simulink model "DC_Motor"  (R2023b)
settings: Solver=VariableStepAuto  StartTime=0.0  StopTime=20  RelTol=1e-3
undefined symbols (not defined in the file): Custom_PID

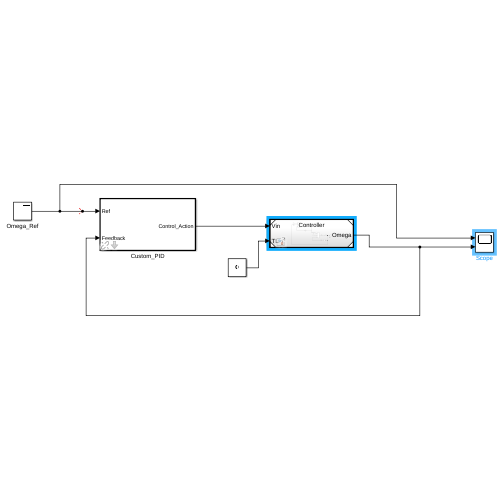
[thumbnail: Simulink's stored preview of the top-level diagram]
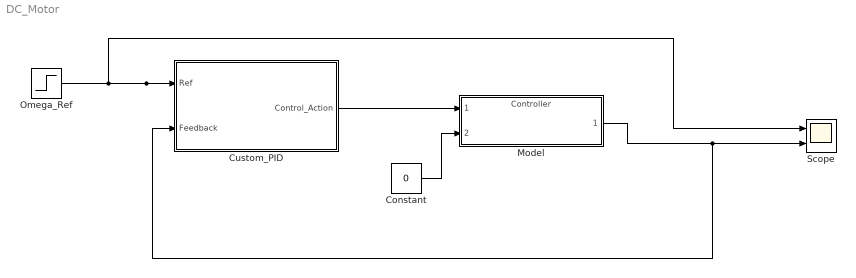
== system DC_Motor ==
  Constant : Constant  Value=0
  Custom_PID : Subsystem  AncestorBlock=Custom_PID/Custom_PID  TreatAsAtomicUnit=on  mask{Kp=8, Ki=2.5, Kd=2, IC=0}
      mask prompts: Kp "Proportional"; Ki "Integral"; Kd "Differential"; IC "Initial Condition"
      mask help:
      | Custom PID Control
      |
      | Propotional is the control Kp
      | Integral is the control Ki
      | Differential is the control Kd
  Model : ModelReference  ModelNameDialog=Controller.slx  SimulationMode=Normal  ModelReferenceVersion=1.4
  Omega_Ref : Step  After=200  SampleTime=0
  Scope : Scope  NumInputPorts=2
  wires:
  Custom_PID/1(Control_Action) -> Model/1
  Omega_Ref/1 -> Custom_PID/1(Ref), Scope/1
  Constant/1 -> Model/2
  Model/1 -> Custom_PID/2(Feedback), Scope/2

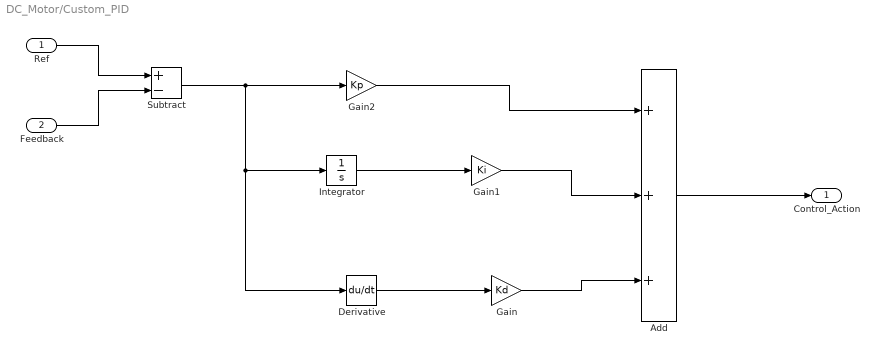
== system DC_Motor/Custom_PID ==
  Ref : Inport
  Feedback : Inport  Port=2
  Add : Sum  Inputs=+++
  Derivative : Derivative
  Gain : Gain  Gain=Kd
  Gain1 : Gain  Gain=Ki
  Gain2 : Gain  Gain=Kp
  Integrator : Integrator  InitialCondition=IC
  Subtract : Sum  Inputs=+-
  Control_Action : Outport
  wires:
  Ref/1 -> Subtract/1
  Add/1 -> Control_Action/1
  Subtract/1 -> Gain2/1, Derivative/1, Integrator/1
  Derivative/1 -> Gain/1
  Feedback/1 -> Subtract/2
  Gain2/1 -> Add/1
  Gain/1 -> Add/3
  Integrator/1 -> Gain1/1
  Gain1/1 -> Add/2
